simulink model "lib_testValidity"  (R2018b)
settings: Solver=VariableStepAuto  StartTime=0.0  StopTime=tfinal  RelTol=1e-3
model workspace (MAT data in the model file):
  q_init = Simulink.Parameter
  q_init.DataType = 'auto'
  q_init.Dimensions = [0 0]
values from neighbouring files (symbols this model uses):
  Bb = Bb./norm(Bb)    [MEKF_ScriptandSimulink_Test.m]    (also in rfrf.m)
  del_t = tspan(2)-tspan(1)    [MEKF_ScriptandSimulink_Test.m]    (also in rfrf.m)
  q = [q(:,2),q(:,3),q(:,4),q(:,1)]    [MEKF_ScriptandSimulink_Test.m]    (also in rfrf.m)
  Ri = Ri./norm(Ri)    [MEKF_ScriptandSimulink_Test.m]    (also in rfrf.m)
undefined symbols (not defined in the file or in its folder): fswParams
libraries: sharedutil x3, dspmtrx3 x2, MEKF_lib x2, aerolibutil x2
settings Model: Creator=kylle  LastModifiedBy=kylle
settings SolverCC: ConsecutiveZCsStepRelTol=0.00001
settings DataIOCC: ReturnWorkspaceOutputs=on  TimeSaveName=timeoutNew  OutputSaveName=youtNew

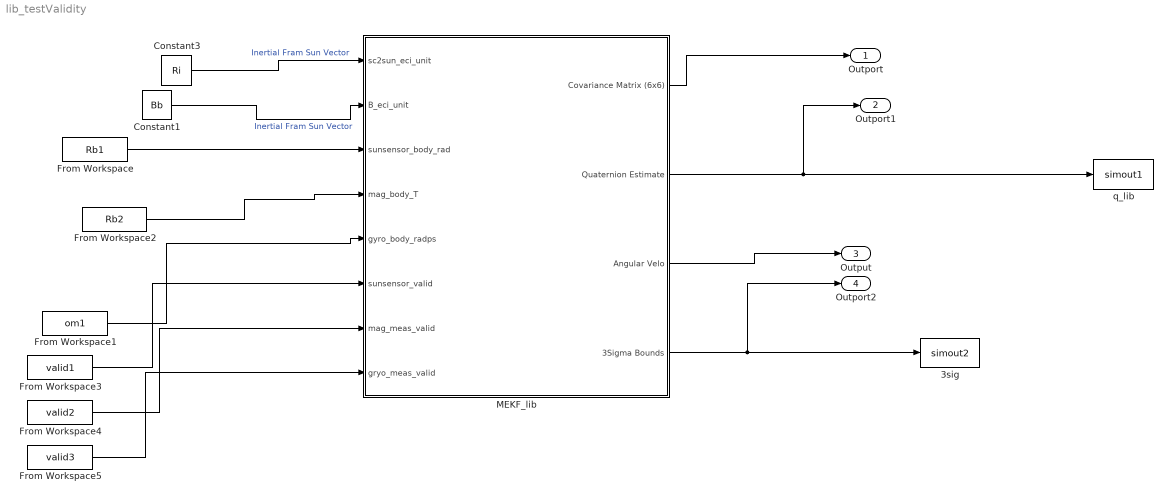
== system lib_testValidity ==
  3sig : ToWorkspace  VariableName=simout2  SaveFormat=Timeseries  SampleTime=-1
  Constant1 : Constant  Value=Bb  VectorParams1D=off
  Constant3 : Constant  Value=Ri  VectorParams1D=off
  From Workspace : FromWorkspace  VariableName=Rb1  SampleTime=del_t
  From Workspace1 : FromWorkspace  VariableName=om1  SampleTime=del_t
  From Workspace2 : FromWorkspace  VariableName=Rb2  SampleTime=del_t
  From Workspace3 : FromWorkspace  VariableName=valid1  SampleTime=del_t
  From Workspace4 : FromWorkspace  VariableName=valid2  SampleTime=del_t
  From Workspace5 : FromWorkspace  VariableName=valid3  SampleTime=del_t
  MEKF_lib : Subsystem  AncestorBlock=MEKF_lib/MEKF_lib
  q_lib : ToWorkspace  VariableName=simout1  SaveFormat=Timeseries  SampleTime=-1
  Outport : Outport
  Outport1 : Outport  Port=2
  Output : Outport  Port=3
  Outport2 : Outport  Port=4
  wires:
  From Workspace1/1 -> MEKF_lib/5(gyro_body_radps)
  MEKF_lib/3("Angular Velo ") -> Output/1
  Constant3/1 -> MEKF_lib/1(sc2sun_eci_unit)  "Inertial Fram Sun Vector"
  MEKF_lib/1(Covariance Matrix (6x6)) -> Outport/1
  Constant1/1 -> MEKF_lib/2(B_eci_unit)  "Inertial Fram Sun Vector"
  From Workspace/1 -> MEKF_lib/3(sunsensor_body_rad)
  From Workspace2/1 -> MEKF_lib/4(mag_body_T)
  From Workspace3/1 -> MEKF_lib/6(sunsensor_valid)
  From Workspace4/1 -> MEKF_lib/7(mag_meas_valid)
  From Workspace5/1 -> MEKF_lib/8(gryo_meas_valid)
  MEKF_lib/2("Quaternion Estimate ") -> q_lib/1, Outport1/1
  MEKF_lib/4("3Sigma Bounds ") -> 3sig/1, Outport2/1

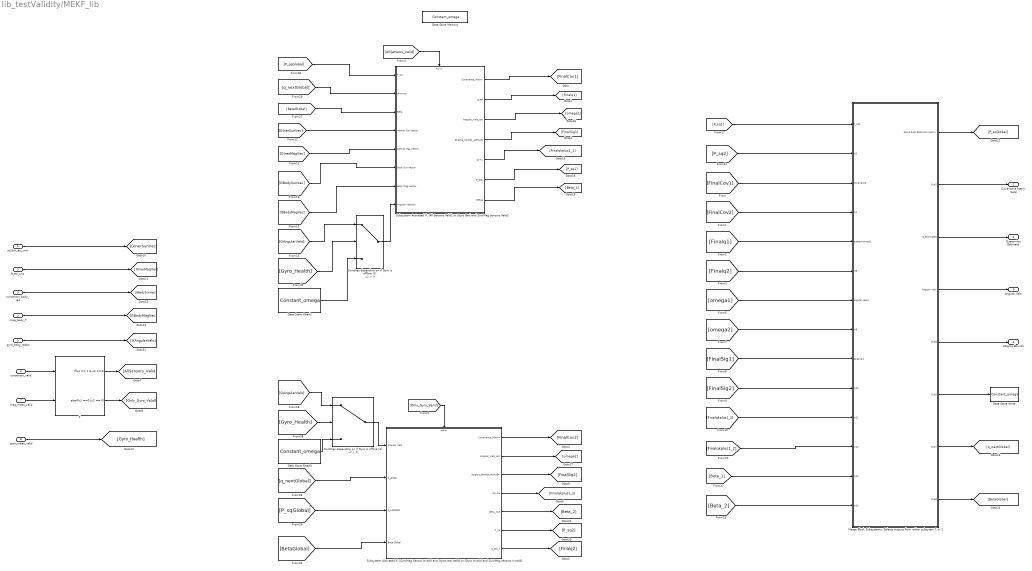
== system lib_testValidity/MEKF_lib ==
  sc2sun_eci_unit : Inport
  B_eci_unit : Inport  Port=2
  sunsensor_body_rad : Inport  Port=3
  mag_body_T : Inport  Port=4
  gyro_body_radps : Inport  Port=5
  sunsensor_valid : Inport  Port=6
  mag_meas_valid : Inport  Port=7
  gryo_meas_valid : Inport  Port=8
  Data Store Memory : DataStoreMemory  DataStoreName=Constant_omega  ReadBeforeWriteMsg=warning  WriteAfterWriteMsg=warning  WriteAfterReadMsg=warning  InitialValue=w0  VectorParams1D=off  ShowAdditionalParam=off
  Data Store Read2 : DataStoreRead  DataStoreName=Constant_omega
  Data Store Read3 : DataStoreRead  DataStoreName=Constant_omega
  Data Store Write : DataStoreWrite  DataStoreName=Constant_omega
  If : If  NumInputs=2  IfExpression=u1 == 1 & u2 ==1  ElseIfExpressions=u1 ==0 |u2 == 0  ShowElse=off
  "Merge Block Subsystems, Selects outputs from either subsytem 1 or 2" : Subsystem
  Subsystem Activated if: [All Sensors Valid] or [Gyro Bad and Sun/Mag sensors Valid] : Subsystem  TreatAsAtomicUnit=on
  Subsystem Activated if: [Sun/Mag Sensor Invalid and Gyros are Valid] or [Gyro Invalid and Sun/Mag sensors Invalid] : Subsystem  TreatAsAtomicUnit=on
  Switches depending on if Gyro is offline (1) : Switch  Criteria=u2 > Threshold
  Switches depending on if Gyro is offline (2) : Switch  Criteria=u2 > Threshold
  Covariance Matrix (6x6) : Outport
  "Quaternion Estimate " : Outport  Port=2
  "Angular Velo " : Outport  Port=3
  "3Sigma Bounds " : Outport  Port=4
  wires:
  [GBodySunVec] -> Subsystem Activated if: [All Sensors Valid] or [Gyro Bad and Sun/Mag sensors Valid]/6(Body Sun Vector)
  [GInerMagVec] -> Subsystem Activated if: [All Sensors Valid] or [Gyro Bad and Sun/Mag sensors Valid]/5(Inertial Mag Vector)
  [GBodyMagVec] -> Subsystem Activated if: [All Sensors Valid] or [Gyro Bad and Sun/Mag sensors Valid]/7(Body Mag Vector)
  Subsystem Activated if: [Sun/Mag Sensor Invalid and Gyros are Valid] or [Gyro Invalid and Sun/Mag sensors Invalid]/4(qk+1a) -> [Finalqkplus1_2]
  Subsystem Activated if: [All Sensors Valid] or [Gyro Bad and Sun/Mag sensors Valid]/2(q_est) -> [Finalq1]
  Subsystem Activated if: [All Sensors Valid] or [Gyro Bad and Sun/Mag sensors Valid]/1(Covariance_Matrix) -> [FinalCov1]
  [Only_Gyro_Valid] -> Subsystem Activated if: [Sun/Mag Sensor Invalid and Gyros are Valid] or [Gyro Invalid and Sun/Mag sensors Invalid]/Action
  Subsystem Activated if: [All Sensors Valid] or [Gyro Bad and Sun/Mag sensors Valid]/4(3sigma_bounds_attitude) -> [FinalSig1]
  Subsystem Activated if: [Sun/Mag Sensor Invalid and Gyros are Valid] or [Gyro Invalid and Sun/Mag sensors Invalid]/7(q_est_k) -> [Finalq2]
  [GInerSunVec] -> Subsystem Activated if: [All Sensors Valid] or [Gyro Bad and Sun/Mag sensors Valid]/4(Inertial Sun Vector)
  Subsystem Activated if: [Sun/Mag Sensor Invalid and Gyros are Valid] or [Gyro Invalid and Sun/Mag sensors Invalid]/1(Covariance_Matrix) -> [FinalCov2]
  [AllSensors_Valid] -> Subsystem Activated if: [All Sensors Valid] or [Gyro Bad and Sun/Mag sensors Valid]/Action
  Subsystem Activated if: [Sun/Mag Sensor Invalid and Gyros are Valid] or [Gyro Invalid and Sun/Mag sensors Invalid]/3(3sigma_bounds_attitude) -> [FinalSig2]
  [q_nextGlobal] -> Subsystem Activated if: [Sun/Mag Sensor Invalid and Gyros are Valid] or [Gyro Invalid and Sun/Mag sensors Invalid]/2(q_global)
  Subsystem Activated if: [All Sensors Valid] or [Gyro Bad and Sun/Mag sensors Valid]/5(qk+1) -> [Finalqkplus1_1]
  [P_sqGlobal] -> Subsystem Activated if: [Sun/Mag Sensor Invalid and Gyros are Valid] or [Gyro Invalid and Sun/Mag sensors Invalid]/3(P_sqGlobal)
  [BetaGlobal] -> Subsystem Activated if: [Sun/Mag Sensor Invalid and Gyros are Valid] or [Gyro Invalid and Sun/Mag sensors Invalid]/4(Beta Global)
  [BetaGlobal] -> Subsystem Activated if: [All Sensors Valid] or [Gyro Bad and Sun/Mag sensors Valid]/3(Beta)
  Subsystem Activated if: [All Sensors Valid] or [Gyro Bad and Sun/Mag sensors Valid]/3(Angular_Velo_est) -> [omega1]
  Subsystem Activated if: [All Sensors Valid] or [Gyro Bad and Sun/Mag sensors Valid]/6("P_Sqa ") -> [P_sq1]
  Subsystem Activated if: [All Sensors Valid] or [Gyro Bad and Sun/Mag sensors Valid]/7(Betaa) -> [Beta_1]
  Subsystem Activated if: [Sun/Mag Sensor Invalid and Gyros are Valid] or [Gyro Invalid and Sun/Mag sensors Invalid]/6(P_sq) -> [P_sq2]
  Subsystem Activated if: [Sun/Mag Sensor Invalid and Gyros are Valid] or [Gyro Invalid and Sun/Mag sensors Invalid]/5(Beta_Out) -> [Beta_2]
  Subsystem Activated if: [Sun/Mag Sensor Invalid and Gyros are Valid] or [Gyro Invalid and Sun/Mag sensors Invalid]/2(Angular_Velo_est) -> [omega2]
  [q_nextGlobal] -> Subsystem Activated if: [All Sensors Valid] or [Gyro Bad and Sun/Mag sensors Valid]/2(qkminus)
  [P_sqGlobal] -> Subsystem Activated if: [All Sensors Valid] or [Gyro Bad and Sun/Mag sensors Valid]/1(P_sq)
  If/1 -> [AllSensors_Valid]
  If/2 -> [Only_Gyro_Valid]
  [GAngularVelo] -> Switches depending on if Gyro is offline (1)/1
  [Gyro_Health] -> Switches depending on if Gyro is offline (1)/2
  Data Store Read2/1 -> Switches depending on if Gyro is offline (1)/3
  Switches depending on if Gyro is offline (1)/1 -> Subsystem Activated if: [All Sensors Valid] or [Gyro Bad and Sun/Mag sensors Valid]/8(Angular Velocity)
  [Gyro_Health] -> Switches depending on if Gyro is offline (2)/2
  [GAngularVelo] -> Switches depending on if Gyro is offline (2)/1
  Data Store Read3/1 -> Switches depending on if Gyro is offline (2)/3
  Switches depending on if Gyro is offline (2)/1 -> Subsystem Activated if: [Sun/Mag Sensor Invalid and Gyros are Valid] or [Gyro Invalid and Sun/Mag sensors Invalid]/1(Angular Velo)
  [P_sq1] -> "Merge Block Subsystems, Selects outputs from either subsytem 1 or 2"/1(P_sq1)
  [P_sq2] -> "Merge Block Subsystems, Selects outputs from either subsytem 1 or 2"/2(In2)
  [FinalCov1] -> "Merge Block Subsystems, Selects outputs from either subsytem 1 or 2"/3(covariance)
  [FinalCov2] -> "Merge Block Subsystems, Selects outputs from either subsytem 1 or 2"/4(In4)
  [Finalq1] -> "Merge Block Subsystems, Selects outputs from either subsytem 1 or 2"/5(quaternion est1)
  [Finalq2] -> "Merge Block Subsystems, Selects outputs from either subsytem 1 or 2"/6(In6)
  [omega1] -> "Merge Block Subsystems, Selects outputs from either subsytem 1 or 2"/7(angular velo1)
  [omega2] -> "Merge Block Subsystems, Selects outputs from either subsytem 1 or 2"/8(In8)
  [FinalSig1] -> "Merge Block Subsystems, Selects outputs from either subsytem 1 or 2"/9(3sigma 1)
  [FinalSig2] -> "Merge Block Subsystems, Selects outputs from either subsytem 1 or 2"/10(In10)
  [Finalqkplus1_1] -> "Merge Block Subsystems, Selects outputs from either subsytem 1 or 2"/11(In11)
  [Finalqkplus1_2] -> "Merge Block Subsystems, Selects outputs from either subsytem 1 or 2"/12(In12)
  [Beta_1] -> "Merge Block Subsystems, Selects outputs from either subsytem 1 or 2"/13(In13)
  [Beta_2] -> "Merge Block Subsystems, Selects outputs from either subsytem 1 or 2"/14(In14)
  "Merge Block Subsystems, Selects outputs from either subsytem 1 or 2"/1(Squre Root State Cov Matrix) -> [P_sqGlobal]
  "Merge Block Subsystems, Selects outputs from either subsytem 1 or 2"/2(Out2) -> Covariance Matrix (6x6)/1
  "Merge Block Subsystems, Selects outputs from either subsytem 1 or 2"/3(q_estimated) -> "Quaternion Estimate "/1
  "Merge Block Subsystems, Selects outputs from either subsytem 1 or 2"/4(Angular Velo) -> "Angular Velo "/1
  "Merge Block Subsystems, Selects outputs from either subsytem 1 or 2"/6(Out5) -> Data Store Write/1
  "Merge Block Subsystems, Selects outputs from either subsytem 1 or 2"/5(Out6) -> "3Sigma Bounds "/1
  "Merge Block Subsystems, Selects outputs from either subsytem 1 or 2"/7(Out7) -> [q_nextGlobal]
  "Merge Block Subsystems, Selects outputs from either subsytem 1 or 2"/8(Out8) -> [BetaGlobal]
  sc2sun_eci_unit/1 -> [GInerSunVec]
  sunsensor_body_rad/1 -> [GBodySunVec]
  sunsensor_valid/1 -> If/1
  mag_meas_valid/1 -> If/2
  gryo_meas_valid/1 -> [Gyro_Health]
  B_eci_unit/1 -> [GInerMagVec]
  mag_body_T/1 -> [GBodyMagVec]
  gyro_body_radps/1 -> [GAngularVelo]

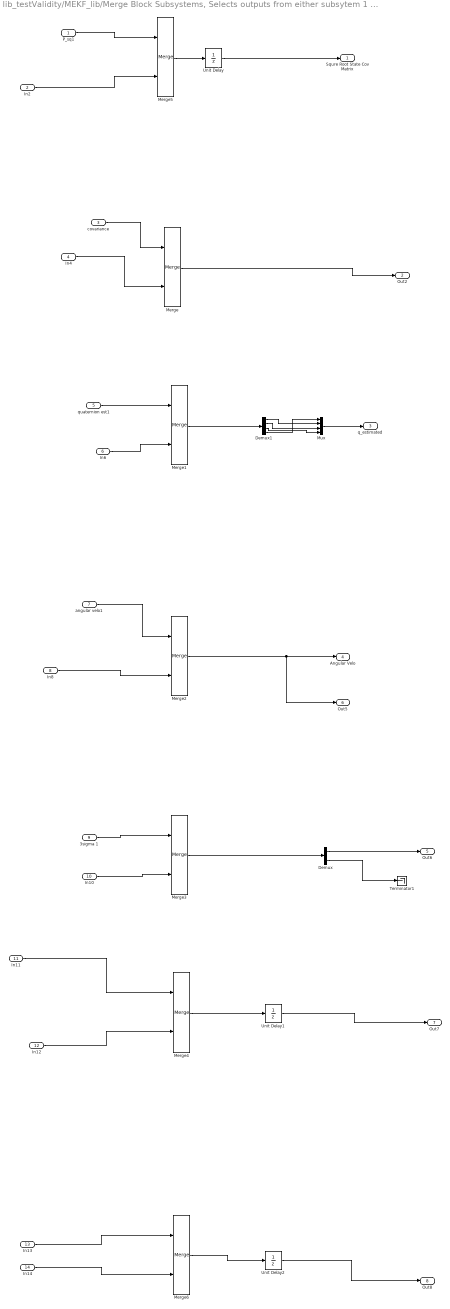
== system lib_testValidity/MEKF_lib/Merge Block Subsystems, Selects outputs from either subsytem 1 or 2 ==
  P_sq1 : Inport
  In2 : Inport  Port=2
  covariance : Inport  Port=3
  In4 : Inport  Port=4
  quaternion est1 : Inport  Port=5
  In6 : Inport  Port=6
  angular velo1 : Inport  Port=7
  In8 : Inport  Port=8
  3sigma 1 : Inport  Port=9
  In10 : Inport  Port=10
  In11 : Inport  Port=11
  In12 : Inport  Port=12
  In13 : Inport  Port=13
  In14 : Inport  Port=14
  Demux : Demux  Outputs=2
  Demux1 : Demux
  Merge{,1..6} (7 alike) : Merge
  Mux : Mux
  Terminator1 : Terminator
  Unit Delay : UnitDelay  InitialCondition=fswParams.estimation.ic.P_sq_init  SampleTime=-1
  Unit Delay1 : UnitDelay  InitialCondition=fswParams.estimation.ic.quat_est_init  SampleTime=-1
  Unit Delay2 : UnitDelay  InitialCondition=fswParams.estimation.ic.Beta_init  SampleTime=-1
  Squre Root State Cov Matrix : Outport
  Out2 : Outport  Port=2
  q_estimated : Outport  Port=3
  Angular Velo : Outport  Port=4
  Out6 : Outport  Port=5
  Out5 : Outport  Port=6
  Out7 : Outport  Port=7
  Out8 : Outport  Port=8
  wires:
  Merge3/1 -> Demux/1
  Merge2/1 -> Out5/1, Angular Velo/1
  Unit Delay1/1 -> Out7/1
  Demux/2 -> Terminator1/1
  Merge6/1 -> Unit Delay2/1
  3sigma 1/1 -> Merge3/1
  quaternion est1/1 -> Merge1/1
  In14/1 -> Merge6/2
  angular velo1/1 -> Merge2/1
  In11/1 -> Merge4/1
  Merge5/1 -> Unit Delay/1
  In10/1 -> Merge3/2
  In2/1 -> Merge5/2
  covariance/1 -> Merge/1
  Merge4/1 -> Unit Delay1/1
  In4/1 -> Merge/2
  Demux/1 -> Out6/1
  In13/1 -> Merge6/1
  Merge/1 -> Out2/1
  In6/1 -> Merge1/2
  In8/1 -> Merge2/2
  In12/1 -> Merge4/2
  P_sq1/1 -> Merge5/1
  Unit Delay2/1 -> Out8/1
  Unit Delay/1 -> Squre Root State Cov Matrix/1
  Merge1/1 -> Demux1/1
  Demux1/4 -> Mux/1
  Demux1/1 -> Mux/2
  Demux1/2 -> Mux/3
  Demux1/3 -> Mux/4
  Mux/1 -> q_estimated/1

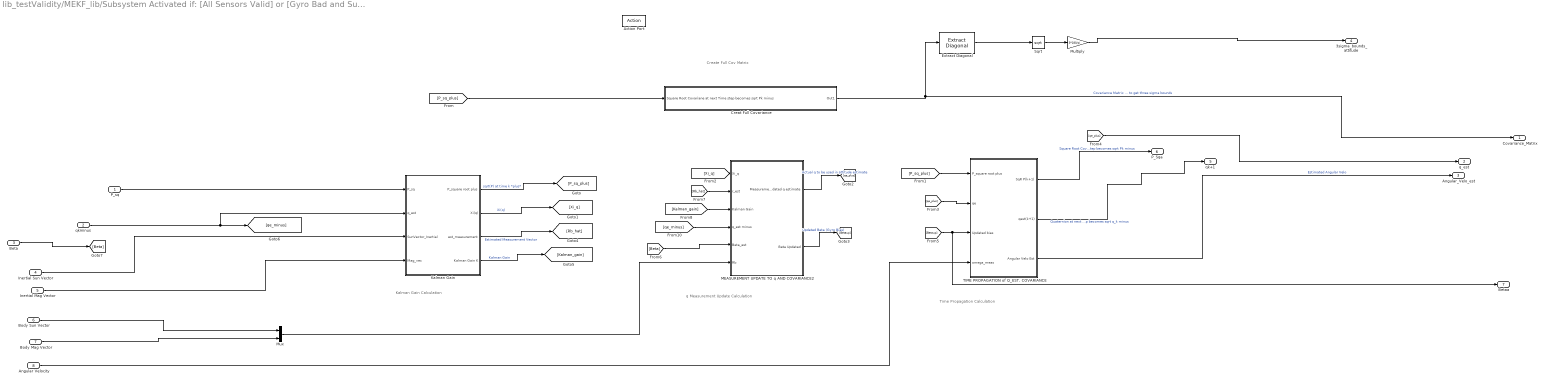
== system lib_testValidity/MEKF_lib/Subsystem Activated if: [All Sensors Valid] or [Gyro Bad and Sun//Mag sensors Valid] ==
  note: Kalman Gain Calculation
  note: Time Propagation Calculation
  note: Create Full Cov Matrix
  note: q Measurement Update Calculation
  P_sq : Inport
  qkminus : Inport  Port=2
  Beta : Inport  Port=3
  Inertial Sun Vector : Inport  Port=4
  Inertial Mag Vector : Inport  Port=5
  Body Sun Vector : Inport  Port=6
  Body Mag Vector : Inport  Port=7
  Angular Velocity : Inport  Port=8
  Action Port : ActionPort  ActionType=then
  Creat Full Covariance : Subsystem  AncestorBlock=MEKF_LibraryR2018b/Multiplicative Extended Kalman Filter/Creat Full Covariance
  Extract Diagonal : dspmtrx3/Extract Diagonal
      settings: SourceProductName=DSP System Toolbox  SourceProductBaseCode=DS
  Kalman Gain : Subsystem  AncestorBlock=MEKF_LibraryR2018b/Multiplicative Extended Kalman Filter/Kalman Gain
  MEASUREMENT UPDATE TO q AND COVARIANCE2 : Subsystem  AncestorBlock=MEKF_LibraryR2018b/Multiplicative Extended Kalman Filter/MEASUREMENT UPDATE TO q AND COVARIANCE2
  Multiply : Gain  Gain=3*180/pi
  Mux : Mux  Inputs=2
  Sqrt : Sqrt  SaturateOnIntegerOverflow=on
  "TIME PROPAGATION of Q_EST, COVARIANCE" : Subsystem  AncestorBlock=MEKF_Library/Multiplicative Extended Kalman Filter/TIME PROPAGATION of Q_EST, COVARIANCE
  Covariance_Matrix : Outport
  q_est : Outport  Port=2
  Angular_Velo_est : Outport  Port=3
  3sigma_bounds_attitude : Outport  Port=4
  qk+1 : Outport  Port=5
  "P_Sqa " : Outport  Port=6
  Betaa : Outport  Port=7
  wires:
  Inertial Sun Vector/1 -> Kalman Gain/3(SunVector_Inertial)
  [qe_plus] -> q_est/1
  "TIME PROPAGATION of Q_EST, COVARIANCE"/2(qest(k+1)) -> qk+1/1  "Quaternion at next Time step becomes sqrt q_k minus"
  "TIME PROPAGATION of Q_EST, COVARIANCE"/3(Angular Velo Est) -> Angular_Velo_est/1  "Estimated Angular Velo"
  Creat Full Covariance/1(Out1) -> Covariance_Matrix/1, Extract Diagonal/1  "Covariance Matrix from which to get three sigma bounds"
  qkminus/1 -> Kalman Gain/2(q_est), [qe_minus]
  Extract Diagonal/1 -> Sqrt/1
  Angular Velocity/1 -> "TIME PROPAGATION of Q_EST, COVARIANCE"/4(omega_meas)
  P_sq/1 -> Kalman Gain/1(P_sq)
  [qe_plus] -> "TIME PROPAGATION of Q_EST, COVARIANCE"/2(qe)
  MEASUREMENT UPDATE TO q AND COVARIANCE2/2(Beta Updated) -> [Betaup]  "Updated Beta (Gyro Bias)"
  [Rb_hat] -> MEASUREMENT UPDATE TO q AND COVARIANCE2/2(r_est)
  "TIME PROPAGATION of Q_EST, COVARIANCE"/1(SqR P(k+1)) -> "P_Sqa "/1  "Square Root Covariane at next Time step becomes sqrt Pk minus"
  Kalman Gain/1(P_square root plus) -> [P_sq_plus]  "sqrt(P) at time k *plus*"
  Kalman Gain/4(Kalman Gain K) -> [Kalman_gain]  "Kalman Gain"
  [qe_minus] -> MEASUREMENT UPDATE TO q AND COVARIANCE2/4(q_est minus)
  Kalman Gain/2(Xi(q)) -> [Xi_q]  "Xi(q)"
  Sqrt/1 -> Multiply/1
  [P_sq_plus] -> Creat Full Covariance/1(Square Root Covariane at next Time step becomes sqrt Pk minus)
  [Betaup] -> Betaa/1, "TIME PROPAGATION of Q_EST, COVARIANCE"/3(Updated bias)
  [Beta] -> MEASUREMENT UPDATE TO q AND COVARIANCE2/5(Beta_est)
  MEASUREMENT UPDATE TO q AND COVARIANCE2/1(Measurement updated q estimate) -> [qe_plus]  "Actual q to be used in attitude estimate"
  [P_sq_plus] -> "TIME PROPAGATION of Q_EST, COVARIANCE"/1(P_square root plus)
  Kalman Gain/3(est_measurement) -> [Rb_hat]  "Estimated Measurement Vector"
  [Xi_q] -> MEASUREMENT UPDATE TO q AND COVARIANCE2/1(Xi_q)
  [Kalman_gain] -> MEASUREMENT UPDATE TO q AND COVARIANCE2/3(Kalman Gain)
  Inertial Mag Vector/1 -> Kalman Gain/4("Mag_vec ")
  Body Sun Vector/1 -> Mux/1
  Body Mag Vector/1 -> Mux/2
  Mux/1 -> MEASUREMENT UPDATE TO q AND COVARIANCE2/6(Rb)
  Multiply/1 -> 3sigma_bounds_attitude/1
  Beta/1 -> [Beta]

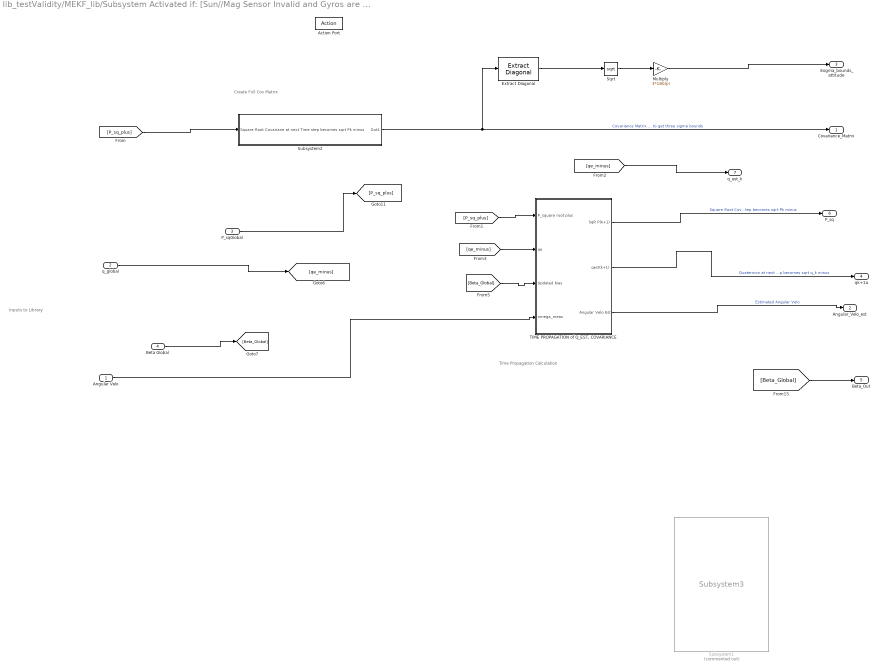
== system lib_testValidity/MEKF_lib/Subsystem Activated if: [Sun//Mag Sensor Invalid and Gyros are Valid] or [Gyro Invalid and Sun//Mag sensors Invalid] ==
  note: Create Full Cov Matrix
  note: Inputs to Library
  note: Time Propagation Calculation
  Angular Velo : Inport
  q_global : Inport  Port=2
  P_sqGlobal : Inport  Port=3
  Beta Global : Inport  Port=4
  Action Port : ActionPort  ActionType=elseif
  Extract Diagonal : dspmtrx3/Extract Diagonal
      settings: SourceProductName=DSP System Toolbox  SourceProductBaseCode=DS
  Multiply : Gain  Gain=3*180/pi
  Sqrt : Sqrt  SaturateOnIntegerOverflow=on
  Subsystem1 : MEKF_lib/MEKF with Validity Check/Subsystem Activated if: [Sun//Mag Sensor Invalid and Gyros are Valid] or [Gyro Invalid and Sun//Mag sensors Invalid]/Subsystem3  Commented=on  SystemSampleTime=-1  SSRTWFcnClass=[]
  Subsystem2 : Subsystem
  "TIME PROPAGATION of Q_EST, COVARIANCE" : Subsystem  AncestorBlock=|
      | MEKF_SensorCheck_Lib2018/MEKF with Validity Check/Subsystem Activated if: [All Sensors Valid]
      | or
      | [Gyro Bad and Sun//Mag sensors Valid]/TIME PROPAGATION of Q_EST, COVARIANCE
  Covariance_Matrix : Outport
  Angular_Velo_est : Outport  Port=2
  3sigma_bounds_attitude : Outport  Port=3
  qk+1a : Outport  Port=4
  Beta_Out : Outport  Port=5
  P_sq : Outport  Port=6
  q_est_k : Outport  Port=7
  wires:
  P_sqGlobal/1 -> [P_sq_plus]
  [qe_minus] -> "TIME PROPAGATION of Q_EST, COVARIANCE"/2(qe)
  "TIME PROPAGATION of Q_EST, COVARIANCE"/2(qest(k+1)) -> qk+1a/1  "Quaternion at next Time step becomes sqrt q_k minus"
  Sqrt/1 -> Multiply/1
  Subsystem2/1(Out1) -> Covariance_Matrix/1, Extract Diagonal/1  "Covariance Matrix from which to get three sigma bounds"
  "TIME PROPAGATION of Q_EST, COVARIANCE"/3(Angular Velo Est) -> Angular_Velo_est/1  "Estimated Angular Velo"
  [P_sq_plus] -> Subsystem2/1(Square Root Covariane at next Time step becomes sqrt Pk minus)
  [P_sq_plus] -> "TIME PROPAGATION of Q_EST, COVARIANCE"/1(P_square root plus)
  [Beta_Global] -> "TIME PROPAGATION of Q_EST, COVARIANCE"/3(Updated bias)
  Extract Diagonal/1 -> Sqrt/1
  q_global/1 -> [qe_minus]
  Angular Velo/1 -> "TIME PROPAGATION of Q_EST, COVARIANCE"/4(omega_meas)
  Multiply/1 -> 3sigma_bounds_attitude/1
  "TIME PROPAGATION of Q_EST, COVARIANCE"/1(SqR P(k+1)) -> P_sq/1  "Square Root Covariane at next Time step becomes sqrt Pk minus"
  Beta Global/1 -> [Beta_Global]
  [Beta_Global] -> Beta_Out/1
  [qe_minus] -> q_est_k/1

== system lib_testValidity/MEKF_lib/Subsystem Activated if: [All Sensors Valid] or [Gyro Bad and Sun//Mag sensors Valid]/Creat Full Covariance ==
  Square Root Covariane at next Time step becomes sqrt Pk minus : Inport
  Matrix Multiply : Product  Multiplication=Matrix(*)
  Transpose : Math  Operator=transpose  SaturateOnIntegerOverflow=on
  Out1 : Outport
  wires:
  Square Root Covariane at next Time step becomes sqrt Pk minus/1 -> Transpose/1, Matrix Multiply/1
  Transpose/1 -> Matrix Multiply/2
  Matrix Multiply/1 -> Out1/1

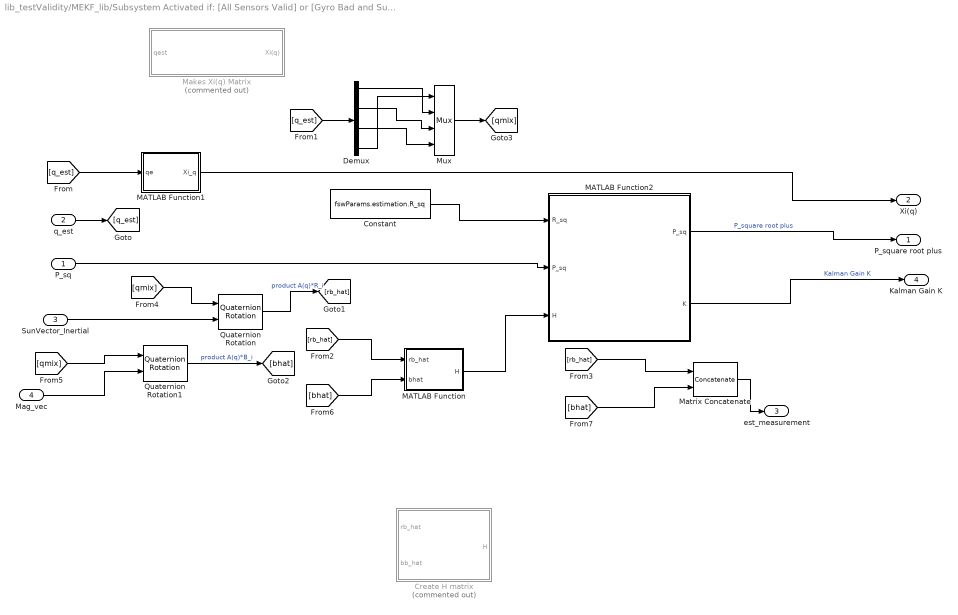
== system lib_testValidity/MEKF_lib/Subsystem Activated if: [All Sensors Valid] or [Gyro Bad and Sun//Mag sensors Valid]/Kalman Gain ==
  P_sq : Inport
  q_est : Inport  Port=2
  SunVector_Inertial : Inport  Port=3
  "Mag_vec " : Inport  Port=4
  Constant : Constant  Value=fswParams.estimation.R_sq  VectorParams1D=off
  Create H matrix : Subsystem  Commented=on
  Demux : Demux
  MATLAB Function : MATLAB Function  TreatAsAtomicUnit=on
  MATLAB Function1 : MATLAB Function  TreatAsAtomicUnit=on
  MATLAB Function2 : MATLAB Function  TreatAsAtomicUnit=on
  Makes Xi(q) Matrix : Subsystem  Commented=on
  Matrix Concatenate : Concatenate  Mode=Multidimensional array
  Mux : Mux
  Quaternion Rotation : aerolibutil/Quaternion Rotation
  Quaternion Rotation1 : aerolibutil/Quaternion Rotation
  P_square root plus : Outport
  Xi(q) : Outport  Port=2
  est_measurement : Outport  Port=3
  Kalman Gain K : Outport  Port=4
  wires:
  P_sq/1 -> MATLAB Function2/2("P_sq ")
  MATLAB Function2/2(K) -> Kalman Gain K/1  "Kalman Gain K"
  SunVector_Inertial/1 -> Quaternion Rotation/2
  Constant/1 -> MATLAB Function2/1(R_sq)
  MATLAB Function2/1(P_sq) -> P_square root plus/1  "P_square root plus"
  Demux/1 -> Mux/2
  Demux/2 -> Mux/3
  Demux/3 -> Mux/4
  Demux/4 -> Mux/1
  q_est/1 -> [q_est]
  [q_est] -> Demux/1
  Quaternion Rotation/1 -> [rb_hat]  "product A(q)*R_i"
  "Mag_vec "/1 -> Quaternion Rotation1/2
  Quaternion Rotation1/1 -> [bhat]  "product A(q)*B_i"
  Mux/1 -> [qmix]
  [qmix] -> Quaternion Rotation1/1
  [qmix] -> Quaternion Rotation/1
  [rb_hat] -> Matrix Concatenate/1
  [bhat] -> Matrix Concatenate/2
  Matrix Concatenate/1 -> est_measurement/1
  [rb_hat] -> MATLAB Function/1(rb_hat)
  [bhat] -> MATLAB Function/2(bhat)
  MATLAB Function/1(H) -> MATLAB Function2/3(H)
  [q_est] -> MATLAB Function1/1(qe)
  MATLAB Function1/1(Xi_q) -> Xi(q)/1

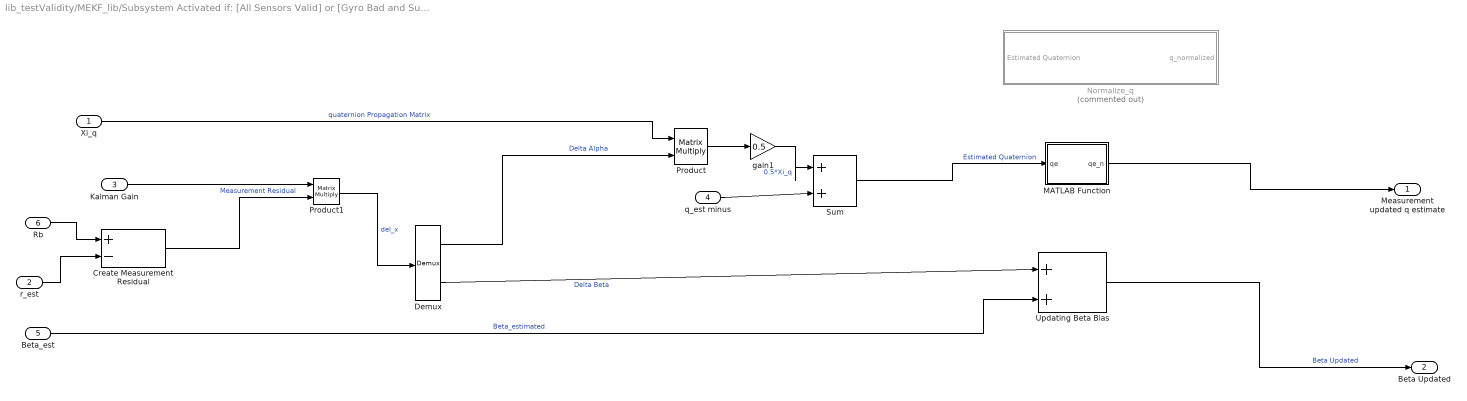
== system lib_testValidity/MEKF_lib/Subsystem Activated if: [All Sensors Valid] or [Gyro Bad and Sun//Mag sensors Valid]/MEASUREMENT UPDATE TO q AND COVARIANCE2 ==
  Xi_q : Inport
  r_est : Inport  Port=2
  Kalman Gain : Inport  Port=3
  q_est minus : Inport  Port=4
  Beta_est : Inport  Port=5
  Rb : Inport  Port=6
  Create Measurement Residual : Sum  Inputs=+-
  Demux : Demux  Outputs=2
  MATLAB Function : MATLAB Function  TreatAsAtomicUnit=on
  Normalize_q : Subsystem  Commented=on
  Product : Product  Inputs=**  Multiplication=Matrix(*)
  Product1 : Product  Multiplication=Matrix(*)
  Sum : Sum  Inputs=|++
  "Updating Beta Bias " : Sum  Inputs=|++
  gain1 : Gain  Gain=0.5
  Measurement updated q estimate : Outport
  Beta Updated : Outport  Port=2
  wires:
  Demux/1 -> Product/2  "Delta Alpha"
  Demux/2 -> "Updating Beta Bias "/1  "Delta Beta"
  Product1/1 -> Demux/1  "del_x"
  r_est/1 -> Create Measurement Residual/2
  Create Measurement Residual/1 -> Product1/2  "Measurement Residual"
  "Updating Beta Bias "/1 -> Beta Updated/1  "Beta Updated"
  Beta_est/1 -> "Updating Beta Bias "/2  "Beta_estimated"
  q_est minus/1 -> Sum/2
  Kalman Gain/1 -> Product1/1
  Rb/1 -> Create Measurement Residual/1
  Xi_q/1 -> Product/1  "quaternion Propagation Matrix"
  Product/1 -> gain1/1
  gain1/1 -> Sum/1  "0.5*Xi_q"
  Sum/1 -> MATLAB Function/1(qe)  "Estimated Quaternion"
  MATLAB Function/1(qe_n) -> Measurement updated q estimate/1

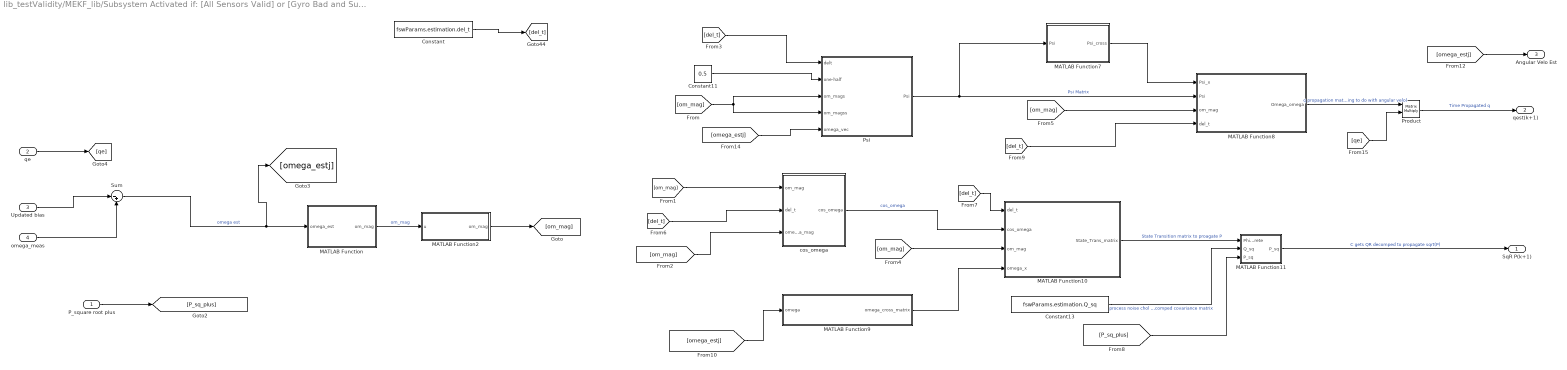
== system lib_testValidity/MEKF_lib/Subsystem Activated if: [All Sensors Valid] or [Gyro Bad and Sun//Mag sensors Valid]/TIME PROPAGATION of Q_EST, COVARIANCE ==
  P_square root plus : Inport
  qe : Inport  Port=2
  Updated bias : Inport  Port=3
  omega_meas : Inport  Port=4
  Constant : Constant  Value=fswParams.estimation.del_t
  Constant11 : Constant  Value=0.5
  Constant13 : Constant  Value=fswParams.estimation.Q_sq  VectorParams1D=off
  MATLAB Function : MATLAB Function  TreatAsAtomicUnit=on
  MATLAB Function10 : MATLAB Function  TreatAsAtomicUnit=on
  MATLAB Function11 : MATLAB Function  TreatAsAtomicUnit=on
  MATLAB Function2 : MATLAB Function  TreatAsAtomicUnit=on
  MATLAB Function7 : MATLAB Function  TreatAsAtomicUnit=on
  MATLAB Function8 : MATLAB Function  TreatAsAtomicUnit=on
  MATLAB Function9 : MATLAB Function  TreatAsAtomicUnit=on
  Product : Product  Multiplication=Matrix(*)
  Psi : Subsystem
  Sum : Sum  Inputs=|-+
  cos_omega : Subsystem
  SqR P(k+1) : Outport
  qest(k+1) : Outport  Port=2
  Angular Velo Est : Outport  Port=3
  wires:
  [del_t] -> MATLAB Function8/4(del_t)
  MATLAB Function7/1(Psi_cross) -> MATLAB Function8/1(Psi_x)
  MATLAB Function11/1(P_sq) -> SqR P(k+1)/1  "C gets QR decomped to propagate sqrt(P)"
  MATLAB Function8/1(Omega_omega) -> Product/1  "q propagation matrix (nothing to do with angular velo)"
  MATLAB Function9/1(omega_cross_matrix) -> MATLAB Function10/4(omega_x)
  MATLAB Function10/1(State_Trans_matrix) -> MATLAB Function11/1(Phi_discrete)  "State Transition matrix to proagate P"
  Product/1 -> qest(k+1)/1  "Time Propagated q"
  Constant13/1 -> MATLAB Function11/2(Q_sq)  "process noise chol decomped covariance matrix"
  omega_meas/1 -> Sum/2
  Updated bias/1 -> Sum/1
  MATLAB Function/1(om_mag) -> MATLAB Function2/1(u)  "om_mag"
  [om_mag] -> MATLAB Function10/3(om_mag)
  [om_mag] -> MATLAB Function8/3(om_mag)
  [del_t] -> MATLAB Function10/1(del_t)
  P_square root plus/1 -> [P_sq_plus]
  [P_sq_plus] -> MATLAB Function11/3("P_sq ")
  [omega_estj] -> MATLAB Function9/1(omega)
  [omega_estj] -> Angular Velo Est/1
  qe/1 -> [qe]
  [qe] -> Product/2
  [om_mag] -> cos_omega/1(om_mag)
  [om_mag] -> cos_omega/3(omega_mag)
  cos_omega/1(cos_omega) -> MATLAB Function10/2(cos_omega)  "cos_omega"
  Psi/1(Psi) -> MATLAB Function8/2(Psi), MATLAB Function7/1(Psi)  "Psi Matrix"
  [del_t] -> Psi/1(delt)
  Constant11/1 -> Psi/2(one-half)
  [omega_estj] -> Psi/5(omega_vec)
  [om_mag] -> Psi/3(om_mags), Psi/4(om_magss)
  Sum/1 -> [omega_estj], MATLAB Function/1(omega_est)  "omega est"
  [del_t] -> cos_omega/2(del_t)
  Constant/1 -> [del_t]
  MATLAB Function2/1(om_mag) -> [om_mag]

== system lib_testValidity/MEKF_lib/Subsystem Activated if: [Sun//Mag Sensor Invalid and Gyros are Valid] or [Gyro Invalid and Sun//Mag sensors Invalid]/Subsystem2 ==
  Square Root Covariane at next Time step becomes sqrt Pk minus : Inport
  Matrix Multiply : Product  Multiplication=Matrix(*)
  Transpose : Math  Operator=transpose  SaturateOnIntegerOverflow=on
  Out1 : Outport
  wires:
  Matrix Multiply/1 -> Out1/1
  Transpose/1 -> Matrix Multiply/2
  Square Root Covariane at next Time step becomes sqrt Pk minus/1 -> Transpose/1, Matrix Multiply/1

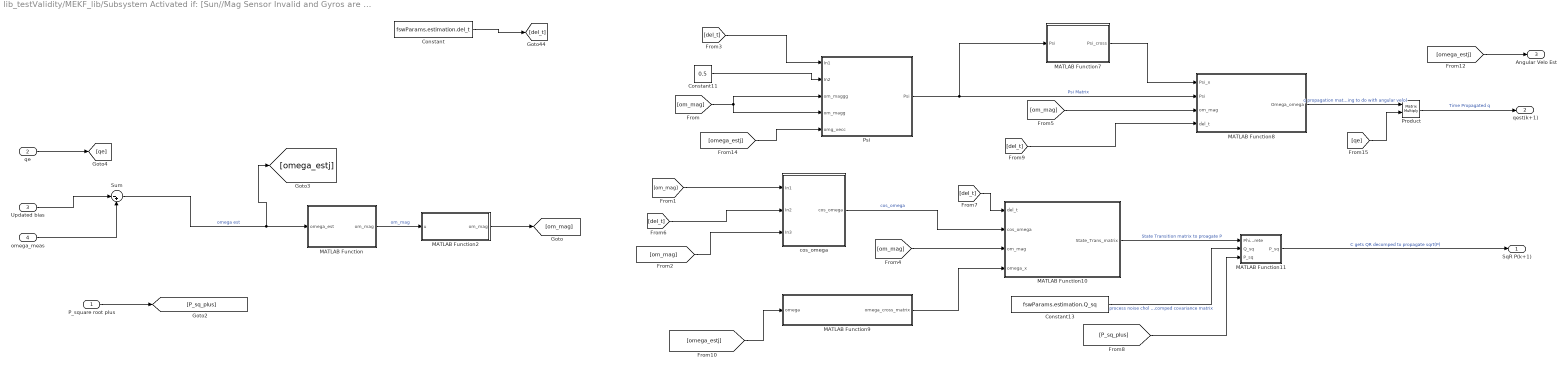
== system lib_testValidity/MEKF_lib/Subsystem Activated if: [Sun//Mag Sensor Invalid and Gyros are Valid] or [Gyro Invalid and Sun//Mag sensors Invalid]/TIME PROPAGATION of Q_EST, COVARIANCE ==
  P_square root plus : Inport
  qe : Inport  Port=2
  Updated bias : Inport  Port=3
  omega_meas : Inport  Port=4
  Constant : Constant  Value=fswParams.estimation.del_t
  Constant11 : Constant  Value=0.5
  Constant13 : Constant  Value=fswParams.estimation.Q_sq  VectorParams1D=off
  MATLAB Function : MATLAB Function  TreatAsAtomicUnit=on
  MATLAB Function10 : MATLAB Function  TreatAsAtomicUnit=on
  MATLAB Function11 : MATLAB Function  TreatAsAtomicUnit=on
  MATLAB Function2 : MATLAB Function  TreatAsAtomicUnit=on
  MATLAB Function7 : MATLAB Function  TreatAsAtomicUnit=on
  MATLAB Function8 : MATLAB Function  TreatAsAtomicUnit=on
  MATLAB Function9 : MATLAB Function  TreatAsAtomicUnit=on
  Product : Product  Multiplication=Matrix(*)
  Psi : Subsystem
  Sum : Sum  Inputs=|-+
  cos_omega : Subsystem
  SqR P(k+1) : Outport
  qest(k+1) : Outport  Port=2
  Angular Velo Est : Outport  Port=3
  wires:
  MATLAB Function2/1(om_mag) -> [om_mag]
  Constant/1 -> [del_t]
  [del_t] -> cos_omega/2(In2)
  Sum/1 -> MATLAB Function/1(omega_est), [omega_estj]  "omega est"
  [om_mag] -> Psi/4(om_magg), Psi/3(om_maggg)
  [omega_estj] -> Psi/5(omg_vecc)
  Constant11/1 -> Psi/2(In2)
  [del_t] -> Psi/1(In1)
  Psi/1(Psi) -> MATLAB Function7/1(Psi), MATLAB Function8/2(Psi)  "Psi Matrix"
  cos_omega/1(cos_omega) -> MATLAB Function10/2(cos_omega)  "cos_omega"
  [om_mag] -> cos_omega/3(In3)
  [om_mag] -> cos_omega/1(In1)
  [qe] -> Product/2
  qe/1 -> [qe]
  [omega_estj] -> Angular Velo Est/1
  [omega_estj] -> MATLAB Function9/1(omega)
  [P_sq_plus] -> MATLAB Function11/3("P_sq ")
  P_square root plus/1 -> [P_sq_plus]
  [del_t] -> MATLAB Function10/1(del_t)
  [om_mag] -> MATLAB Function8/3(om_mag)
  [om_mag] -> MATLAB Function10/3(om_mag)
  MATLAB Function/1(om_mag) -> MATLAB Function2/1(u)  "om_mag"
  Updated bias/1 -> Sum/1
  omega_meas/1 -> Sum/2
  Constant13/1 -> MATLAB Function11/2(Q_sq)  "process noise chol decomped covariance matrix"
  Product/1 -> qest(k+1)/1  "Time Propagated q"
  MATLAB Function10/1(State_Trans_matrix) -> MATLAB Function11/1(Phi_discrete)  "State Transition matrix to proagate P"
  MATLAB Function9/1(omega_cross_matrix) -> MATLAB Function10/4(omega_x)
  MATLAB Function8/1(Omega_omega) -> Product/1  "q propagation matrix (nothing to do with angular velo)"
  MATLAB Function11/1(P_sq) -> SqR P(k+1)/1  "C gets QR decomped to propagate sqrt(P)"
  MATLAB Function7/1(Psi_cross) -> MATLAB Function8/1(Psi_x)
  [del_t] -> MATLAB Function8/4(del_t)

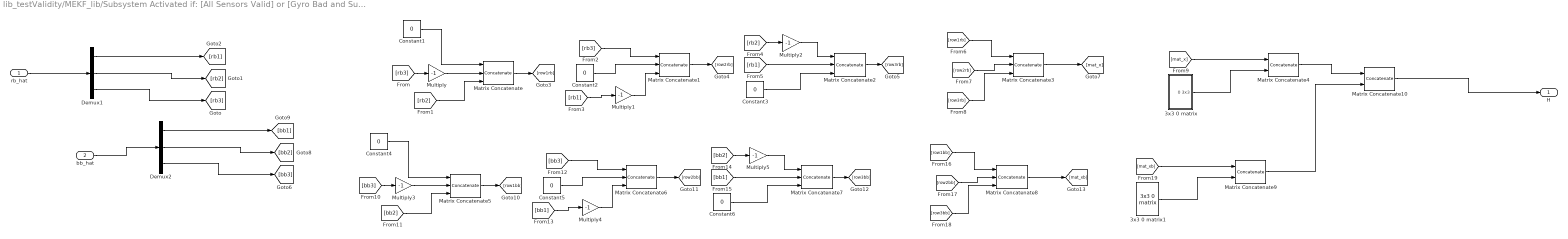
== system lib_testValidity/MEKF_lib/Subsystem Activated if: [All Sensors Valid] or [Gyro Bad and Sun//Mag sensors Valid]/Kalman Gain/Create H matrix ==
  rb_hat : Inport
  bb_hat : Inport  Port=2
  3x3 0 matrix : Subsystem
  3x3 0 matrix1 : MEKF_lib/MEKF_lib/Subsystem Activated if: [All Sensors Valid] or [Gyro Bad and Sun//Mag sensors Valid]/Kalman Gain/Create H matrix/3x3 0 matrix  SystemSampleTime=-1
  Constant{1..6} (6 alike) : Constant  Value=0
  Demux1 : Demux  Outputs=3
  Demux2 : Demux  Outputs=3
  Matrix Concatenate{,1..2,5..7} (6 alike) : Concatenate  NumInputs=3  Mode=Multidimensional array  ConcatenateDimension=2
  Matrix Concatenate10 : Concatenate  Mode=Multidimensional array
  Matrix Concatenate3 : Concatenate  NumInputs=3  Mode=Multidimensional array
  Matrix Concatenate4 : Concatenate  Mode=Multidimensional array  ConcatenateDimension=2
  Matrix Concatenate8 : Concatenate  NumInputs=3  Mode=Multidimensional array
  Matrix Concatenate9 : Concatenate  Mode=Multidimensional array  ConcatenateDimension=2
  Multiply{,1..5} (6 alike) : Gain  Gain=-1
  H : Outport
  wires:
  Matrix Concatenate1/1 -> [row2rb]
  Multiply/1 -> Matrix Concatenate/2
  [mat_x] -> Matrix Concatenate4/1
  Demux1/2 -> [rb2]
  Multiply2/1 -> Matrix Concatenate2/1
  [row3rb] -> Matrix Concatenate3/3
  Matrix Concatenate/1 -> [row1rb]
  Matrix Concatenate2/1 -> [row3rb]
  [rb1] -> Multiply1/1
  [rb3] -> Multiply/1
  Multiply1/1 -> Matrix Concatenate1/3
  Constant3/1 -> Matrix Concatenate2/3
  3x3 0 matrix/1(0 3x3) -> Matrix Concatenate4/2
  [rb2] -> Multiply2/1
  [rb2] -> Matrix Concatenate/3
  [rb3] -> Matrix Concatenate1/1
  [row2rb] -> Matrix Concatenate3/2
  Constant1/1 -> Matrix Concatenate/1
  [row1rb] -> Matrix Concatenate3/1
  Demux1/1 -> [rb1]
  Matrix Concatenate3/1 -> [mat_x]
  Constant2/1 -> Matrix Concatenate1/2
  [rb1] -> Matrix Concatenate2/2
  Demux1/3 -> [rb3]
  rb_hat/1 -> Demux1/1
  Demux2/3 -> [bb3]
  bb_hat/1 -> Demux2/1
  Demux2/1 -> [bb1]
  Demux2/2 -> [bb2]
  Multiply5/1 -> Matrix Concatenate7/1
  [bb1] -> Matrix Concatenate7/2
  Constant4/1 -> Matrix Concatenate5/1
  Multiply3/1 -> Matrix Concatenate5/2
  Constant5/1 -> Matrix Concatenate6/2
  Multiply4/1 -> Matrix Concatenate6/3
  Matrix Concatenate5/1 -> [row1bb]
  [bb1] -> Multiply4/1
  Matrix Concatenate7/1 -> [row3bb]
  Constant6/1 -> Matrix Concatenate7/3
  [bb2] -> Matrix Concatenate5/3
  [bb3] -> Multiply3/1
  [bb3] -> Matrix Concatenate6/1
  [bb2] -> Multiply5/1
  Matrix Concatenate6/1 -> [row2bb]
  [row1bb] -> Matrix Concatenate8/1
  Matrix Concatenate8/1 -> [mat_xb]
  [row2bb] -> Matrix Concatenate8/2
  [row3bb] -> Matrix Concatenate8/3
  3x3 0 matrix1/1 -> Matrix Concatenate9/2
  Matrix Concatenate9/1 -> Matrix Concatenate10/2
  [mat_xb] -> Matrix Concatenate9/1
  Matrix Concatenate4/1 -> Matrix Concatenate10/1
  Matrix Concatenate10/1 -> H/1

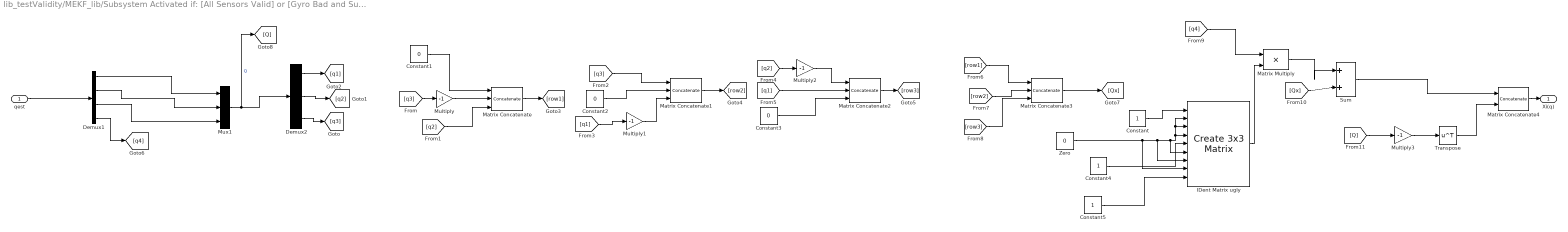
== system lib_testValidity/MEKF_lib/Subsystem Activated if: [All Sensors Valid] or [Gyro Bad and Sun//Mag sensors Valid]/Kalman Gain/Makes Xi(q) Matrix ==
  qest : Inport
  Constant : Constant
  Constant1 : Constant  Value=0
  Constant2 : Constant  Value=0
  Constant3 : Constant  Value=0
  Constant4 : Constant
  Constant5 : Constant
  Demux1 : Demux
  Demux2 : Demux  Outputs=3
  IDent Matrix ugly : sharedutil/Create 3x3 Matrix  aMode=aMode
  Matrix Concatenate : Concatenate  NumInputs=3  Mode=Multidimensional array  ConcatenateDimension=2
  Matrix Concatenate1 : Concatenate  NumInputs=3  Mode=Multidimensional array  ConcatenateDimension=2
  Matrix Concatenate2 : Concatenate  NumInputs=3  Mode=Multidimensional array  ConcatenateDimension=2
  Matrix Concatenate3 : Concatenate  NumInputs=3  Mode=Multidimensional array
  Matrix Concatenate4 : Concatenate  Mode=Multidimensional array
  Matrix Multiply : Product  Inputs=**
  Multiply{,1..3} (4 alike) : Gain  Gain=-1
  Mux1 : Mux  Inputs=3
  Sum : Sum  Inputs=|++
  Transpose : Math  Operator=transpose  SaturateOnIntegerOverflow=on
  Zero : Constant  Value=0  OutDataTypeStr=Inherit: Inherit via back propagation
  Xi(q) : Outport
  wires:
  Multiply2/1 -> Matrix Concatenate2/1
  [q1] -> Matrix Concatenate2/2
  Matrix Multiply/1 -> Sum/1
  Matrix Concatenate1/1 -> [row2]
  Constant1/1 -> Matrix Concatenate/1
  Matrix Concatenate3/1 -> [Qx]
  [q2] -> Matrix Concatenate/3
  Mux1/1 -> Demux2/1, [Q]  "Q"
  Constant2/1 -> Matrix Concatenate1/2
  Demux1/2 -> Mux1/2
  [row3] -> Matrix Concatenate3/3
  qest/1 -> Demux1/1
  Multiply3/1 -> Transpose/1
  [q4] -> Matrix Multiply/1
  [q3] -> Matrix Concatenate1/1
  Demux2/2 -> [q2]
  Sum/1 -> Matrix Concatenate4/1
  [q2] -> Multiply2/1
  Demux1/4 -> [q4]
  [row2] -> Matrix Concatenate3/2
  Demux1/1 -> Mux1/1
  Demux1/3 -> Mux1/3
  Matrix Concatenate2/1 -> [row3]
  [Qx] -> Sum/2
  Multiply/1 -> Matrix Concatenate/2
  [row1] -> Matrix Concatenate3/1
  [Q] -> Multiply3/1
  Demux2/1 -> [q1]
  Transpose/1 -> Matrix Concatenate4/2
  IDent Matrix ugly/1 -> Matrix Multiply/2
  [q3] -> Multiply/1
  Matrix Concatenate/1 -> [row1]
  Demux2/3 -> [q3]
  Constant3/1 -> Matrix Concatenate2/3
  [q1] -> Multiply1/1
  Multiply1/1 -> Matrix Concatenate1/3
  Matrix Concatenate4/1 -> Xi(q)/1
  Constant/1 -> IDent Matrix ugly/1
  Constant5/1 -> IDent Matrix ugly/9
  Constant4/1 -> IDent Matrix ugly/5
  Zero/1 -> IDent Matrix ugly/8, IDent Matrix ugly/7, IDent Matrix ugly/6, IDent Matrix ugly/4, IDent Matrix ugly/3, IDent Matrix ugly/2

== system lib_testValidity/MEKF_lib/Subsystem Activated if: [All Sensors Valid] or [Gyro Bad and Sun//Mag sensors Valid]/MEASUREMENT UPDATE TO q AND COVARIANCE2/Normalize_q ==
  note: Rearrange_Quat
  note: Rearrange_Quat_back
  Estimated Quaternion : Inport
  Demux : Demux
  Demux1 : Demux
  Mux : Mux
  Mux1 : Mux
  Quaternion Normalize : sharedutil/Quaternion Normalize  aMode=aMode
      settings: SourceProductName=Aerospace Blockset  SourceProductBaseCode=AE
  q_normalized : Outport
  wires:
  Mux1/1 -> Quaternion Normalize/1
  Demux1/4 -> Mux1/1
  Demux/4 -> Mux/3
  Demux/3 -> Mux/2
  Demux/2 -> Mux/1
  Demux1/3 -> Mux1/4
  Mux/1 -> q_normalized/1
  Demux1/1 -> Mux1/2
  Demux1/2 -> Mux1/3
  Demux/1 -> Mux/4
  Quaternion Normalize/1 -> Demux/1  "Measurement updated q estimate"
  Estimated Quaternion/1 -> Demux1/1

== system lib_testValidity/MEKF_lib/Subsystem Activated if: [All Sensors Valid] or [Gyro Bad and Sun//Mag sensors Valid]/TIME PROPAGATION of Q_EST, COVARIANCE/Psi ==
  delt : Inport
  one-half : Inport  Port=2
  om_mags : Inport  Port=3
  om_magss : Inport  Port=4
  omega_vec : Inport  Port=5
  Divide : Product  Inputs=***
  Divide1 : Product  Inputs=**/
  Sin : Trigonometry
  Psi : Outport
  wires:
  delt/1 -> Divide/1
  Divide/1 -> Sin/1  "om_mag times0.5*del_t"
  Divide1/1 -> Psi/1  "Psi"
  om_mags/1 -> Divide/3
  Sin/1 -> Divide1/1  "sin(om_mag*0.5*del_t)"
  one-half/1 -> Divide/2
  omega_vec/1 -> Divide1/2
  om_magss/1 -> Divide1/3

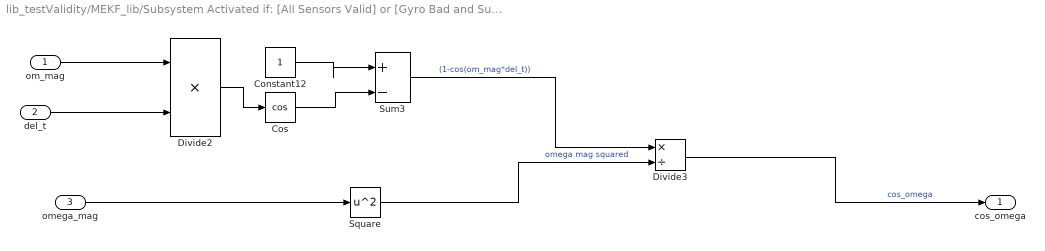
== system lib_testValidity/MEKF_lib/Subsystem Activated if: [All Sensors Valid] or [Gyro Bad and Sun//Mag sensors Valid]/TIME PROPAGATION of Q_EST, COVARIANCE/cos_omega ==
  om_mag : Inport
  del_t : Inport  Port=2
  omega_mag : Inport  Port=3
  Constant12 : Constant
  Cos : Trigonometry  Operator=cos
  Divide2 : Product  Inputs=**
  Divide3 : Product  Inputs=*/
  Square : Math  Operator=square  SaturateOnIntegerOverflow=on
  Sum3 : Sum  Inputs=|+-
  cos_omega : Outport
  wires:
  Divide2/1 -> Cos/1
  omega_mag/1 -> Square/1
  Divide3/1 -> cos_omega/1  "cos_omega"
  Constant12/1 -> Sum3/1
  Square/1 -> Divide3/2  "omega mag squared"
  om_mag/1 -> Divide2/1
  Cos/1 -> Sum3/2
  del_t/1 -> Divide2/2
  Sum3/1 -> Divide3/1  "(1-cos(om_mag*del_t))"

== system lib_testValidity/MEKF_lib/Subsystem Activated if: [Sun//Mag Sensor Invalid and Gyros are Valid] or [Gyro Invalid and Sun//Mag sensors Invalid]/TIME PROPAGATION of Q_EST, COVARIANCE/Psi ==
  In1 : Inport
  In2 : Inport  Port=2
  om_maggg : Inport  Port=3
  om_magg : Inport  Port=4
  omg_vecc : Inport  Port=5
  Divide : Product  Inputs=***
  Divide1 : Product  Inputs=**/
  Sin : Trigonometry
  Psi : Outport
  wires:
  In2/1 -> Divide/2
  Sin/1 -> Divide1/1  "sin(om_mag*0.5*del_t)"
  om_maggg/1 -> Divide/3
  Divide1/1 -> Psi/1  "Psi"
  omg_vecc/1 -> Divide1/2
  om_magg/1 -> Divide1/3
  Divide/1 -> Sin/1  "om_mag times0.5*del_t"
  In1/1 -> Divide/1

== system lib_testValidity/MEKF_lib/Subsystem Activated if: [Sun//Mag Sensor Invalid and Gyros are Valid] or [Gyro Invalid and Sun//Mag sensors Invalid]/TIME PROPAGATION of Q_EST, COVARIANCE/cos_omega ==
  In1 : Inport
  In2 : Inport  Port=2
  In3 : Inport  Port=3
  Constant12 : Constant
  Cos : Trigonometry  Operator=cos
  Divide2 : Product  Inputs=**
  Divide3 : Product  Inputs=*/
  Square : Math  Operator=square  SaturateOnIntegerOverflow=on
  Sum3 : Sum  Inputs=|+-
  cos_omega : Outport
  wires:
  Sum3/1 -> Divide3/1  "(1-cos(om_mag*del_t))"
  In2/1 -> Divide2/2
  Cos/1 -> Sum3/2
  In1/1 -> Divide2/1
  Square/1 -> Divide3/2  "omega mag squared"
  Constant12/1 -> Sum3/1
  Divide3/1 -> cos_omega/1  "cos_omega"
  In3/1 -> Square/1
  Divide2/1 -> Cos/1

== system lib_testValidity/MEKF_lib/Subsystem Activated if: [All Sensors Valid] or [Gyro Bad and Sun//Mag sensors Valid]/Kalman Gain/Create H matrix/3x3 0 matrix ==
  Create 3x3 Matrix : sharedutil/Create 3x3 Matrix  aMode=aMode
  Zero : Constant  Value=0  OutDataTypeStr=Inherit: Inherit via back propagation
  0 3x3 : Outport
  wires:
  Zero/1 -> Create 3x3 Matrix/9, Create 3x3 Matrix/8, Create 3x3 Matrix/7, Create 3x3 Matrix/6, Create 3x3 Matrix/1, Create 3x3 Matrix/5, Create 3x3 Matrix/2, Create 3x3 Matrix/3, Create 3x3 Matrix/4
  Create 3x3 Matrix/1 -> 0 3x3/1

== matlab function lib_testValidity/MEKF_lib/Subsystem Activated if: [Sun//Mag Sensor Invalid and Gyros are Valid] or [Gyro Invalid and Sun//Mag sensors Invalid]/TIME PROPAGATION of Q_EST, COVARIANCE/MATLAB Function ==
  data: omega_est input; om_mag output
function om_mag = om2_norm(omega_est)

om_mag = norm(omega_est);

== matlab function lib_testValidity/MEKF_lib/Subsystem Activated if: [Sun//Mag Sensor Invalid and Gyros are Valid] or [Gyro Invalid and Sun//Mag sensors Invalid]/TIME PROPAGATION of Q_EST, COVARIANCE/MATLAB Function10 ==
  data: del_t input; cos_omega input; om_mag input; omega_x input; State_Trans_matrix output
function State_Trans_matrix = Phi_disc(del_t,cos_omega,om_mag,omega_x)
%#codegen

State_Trans_matrix = [(eye(3)-omega_x*sin(om_mag*del_t)/om_mag + (omega_x^2)*cos_omega),omega_x*cos_omega-eye(3)*del_t-omega_x^2*(om_mag*del_t-sin(om_mag*del_t))/om_mag^3;
            zeros(3,3),eye(3)];

== matlab function lib_testValidity/MEKF_lib/Subsystem Activated if: [All Sensors Valid] or [Gyro Bad and Sun//Mag sensors Valid]/Kalman Gain/MATLAB Function2 ==
  data: R_sq input; P_sq input; H input; P_sq output; K output
function [P_sq,K] = fcnAQR(R_sq,P_sq,H)
%#codegen
[nr,mr] = size(R_sq);
[np,mp] = size(P_sq);
% A_QR = [R_sq',zeros(nr,np);(P_sq')*H', P_sq'];
A_QR = [R_sq',zeros(nr,np);(P_sq')*H', P_sq];
[TA,UA] = qr(A_QR);
        P_sq = UA(7:12,7:12)'; %Updated P_sq
        W = UA(1:6,7:12)';
%        
        sq_Bk = UA(1:6,1:6)';
K = W*inv(sq_Bk);

== matlab function lib_testValidity/MEKF_lib/Subsystem Activated if: [Sun//Mag Sensor Invalid and Gyros are Valid] or [Gyro Invalid and Sun//Mag sensors Invalid]/TIME PROPAGATION of Q_EST, COVARIANCE/MATLAB Function11 ==
  data: Phi_discrete input; P_sq output; Q_sq input; P_sq input
function P_sq  = Cqr(Phi_discrete,Q_sq,P_sq)
%#codegen

C = [P_sq'*Phi_discrete';Q_sq'];
          [Tc,Uc] = qr(C);
%           Uc = full(Uc);
          sq_P_kp1 = Uc(1:6,1:6)';
%           P = sq_P_kp1'*sq_P_kp1;
          P_sq = sq_P_kp1;

== matlab function lib_testValidity/MEKF_lib/Subsystem Activated if: [Sun//Mag Sensor Invalid and Gyros are Valid] or [Gyro Invalid and Sun//Mag sensors Invalid]/TIME PROPAGATION of Q_EST, COVARIANCE/MATLAB Function2 ==
  data: u input; om_mag output
function om_mag = norm_check1(u)
%#codegen
if u == 0
    om_mag = 10^-10;
else
    om_mag = u;
end

end

== matlab function lib_testValidity/MEKF_lib/Subsystem Activated if: [Sun//Mag Sensor Invalid and Gyros are Valid] or [Gyro Invalid and Sun//Mag sensors Invalid]/TIME PROPAGATION of Q_EST, COVARIANCE/MATLAB Function7 ==
  data: Psi input; Psi_cross output
function Psi_cross = Psi_cross_matrix(Psi)
%#codegen

Psi_cross = [0 -Psi(3) Psi(2);Psi(3) 0 -Psi(1);-Psi(2) Psi(1) 0];

== matlab function lib_testValidity/MEKF_lib/Subsystem Activated if: [Sun//Mag Sensor Invalid and Gyros are Valid] or [Gyro Invalid and Sun//Mag sensors Invalid]/TIME PROPAGATION of Q_EST, COVARIANCE/MATLAB Function8 ==
  data: Psi_x input; Psi input; om_mag input; del_t input; Omega_omega output
function Omega_omega = omega_omega_matrix(Psi_x,Psi,om_mag,del_t)
%#codegen

 Omega_omega = [(cos(0.5*om_mag*del_t)*eye(3) - Psi_x), Psi; -Psi', cos(0.5*om_mag*del_t)];

== matlab function lib_testValidity/MEKF_lib/Subsystem Activated if: [All Sensors Valid] or [Gyro Bad and Sun//Mag sensors Valid]/TIME PROPAGATION of Q_EST, COVARIANCE/MATLAB Function7 ==
  data: Psi input; Psi_cross output
function Psi_cross = Psi_cross_matrix(Psi)
%#codegen

Psi_cross = [0 -Psi(3) Psi(2);Psi(3) 0 -Psi(1);-Psi(2) Psi(1) 0];

== matlab function lib_testValidity/MEKF_lib/Subsystem Activated if: [All Sensors Valid] or [Gyro Bad and Sun//Mag sensors Valid]/TIME PROPAGATION of Q_EST, COVARIANCE/MATLAB Function8 ==
  data: Psi_x input; Psi input; om_mag input; del_t input; Omega_omega output
function Omega_omega = omega_omega_matrix(Psi_x,Psi,om_mag,del_t)
%#codegen

 Omega_omega = [(cos(0.5*om_mag*del_t)*eye(3) - Psi_x), Psi; -Psi', cos(0.5*om_mag*del_t)];

== matlab function lib_testValidity/MEKF_lib/Subsystem Activated if: [All Sensors Valid] or [Gyro Bad and Sun//Mag sensors Valid]/TIME PROPAGATION of Q_EST, COVARIANCE/MATLAB Function9 ==
  data: omega input; omega_cross_matrix output
function omega_cross_matrix = makes_omega_cross_matrix(omega)

omega_cross_matrix = [0 -omega(3) omega(2);omega(3) 0 -omega(1);-omega(2) omega(1) 0];

== matlab function lib_testValidity/MEKF_lib/Subsystem Activated if: [All Sensors Valid] or [Gyro Bad and Sun//Mag sensors Valid]/TIME PROPAGATION of Q_EST, COVARIANCE/MATLAB Function10 ==
  data: del_t input; cos_omega input; om_mag input; omega_x input; State_Trans_matrix output
function State_Trans_matrix = Phi_disc(del_t,cos_omega,om_mag,omega_x)
%#codegen

State_Trans_matrix = [(eye(3)-omega_x*sin(om_mag*del_t)/om_mag + (omega_x^2)*cos_omega),...
    omega_x*cos_omega-eye(3)*del_t-omega_x^2*(om_mag*del_t-sin(om_mag*del_t))/om_mag^3;
            zeros(3,3),eye(3)];

== matlab function lib_testValidity/MEKF_lib/Subsystem Activated if: [All Sensors Valid] or [Gyro Bad and Sun//Mag sensors Valid]/TIME PROPAGATION of Q_EST, COVARIANCE/MATLAB Function11 ==
  data: Phi_discrete input; P_sq output; Q_sq input; P_sq input
function P_sq  = Cqr(Phi_discrete,Q_sq,P_sq)
%#codegen

C = [P_sq'*Phi_discrete';Q_sq'];
          [Tc,Uc] = qr(C);
%           Uc = full(Uc);
          sq_P_kp1 = Uc(1:6,1:6)';
%           P = sq_P_kp1'*sq_P_kp1;
          P_sq = sq_P_kp1;

== matlab function lib_testValidity/MEKF_lib/Subsystem Activated if: [Sun//Mag Sensor Invalid and Gyros are Valid] or [Gyro Invalid and Sun//Mag sensors Invalid]/TIME PROPAGATION of Q_EST, COVARIANCE/MATLAB Function9 ==
  data: omega input; omega_cross_matrix output
function omega_cross_matrix = makes_omega_cross_matrix(omega)

omega_cross_matrix = [0 -omega(3) omega(2);omega(3) 0 -omega(1);-omega(2) omega(1) 0];

== matlab function lib_testValidity/MEKF_lib/Subsystem Activated if: [All Sensors Valid] or [Gyro Bad and Sun//Mag sensors Valid]/MEASUREMENT UPDATE TO q AND COVARIANCE2/MATLAB Function ==
  data: qe input; qe_n output
function qe_n = fcn(qe)
%#codegen

qe_n = 1/(norm(qe))*qe;

== matlab function lib_testValidity/MEKF_lib/Subsystem Activated if: [All Sensors Valid] or [Gyro Bad and Sun//Mag sensors Valid]/TIME PROPAGATION of Q_EST, COVARIANCE/MATLAB Function ==
  data: omega_est input; om_mag output
function om_mag = om2_norm(omega_est)

om_mag = norm(omega_est);

== matlab function lib_testValidity/MEKF_lib/Subsystem Activated if: [All Sensors Valid] or [Gyro Bad and Sun//Mag sensors Valid]/Kalman Gain/MATLAB Function ==
  data: rb_hat input; H output size=[6,6]; bhat input
function H  = fcn(rb_hat,bhat)
%#codegen

            mat_x = [0 -rb_hat(3) rb_hat(2);rb_hat(3) 0 -rb_hat(1);-rb_hat(2) rb_hat(1) 0]; %cross product matrix of q
            mat_x1 = [0 -bhat(3) bhat(2);bhat(3) 0 -bhat(1);-bhat(2) bhat(1) 0];
        
%%%%% Calcualte Kalman Gain
        H = [mat_x, zeros(3,3);mat_x1,zeros(3,3)]; %sensitivity matrix'

== matlab function lib_testValidity/MEKF_lib/Subsystem Activated if: [All Sensors Valid] or [Gyro Bad and Sun//Mag sensors Valid]/TIME PROPAGATION of Q_EST, COVARIANCE/MATLAB Function2 ==
  data: u input; om_mag output
function om_mag = norm_check1(u)
%#codegen
if u == 0
    om_mag = 10^-10;
else
    om_mag = u;
end
end

== matlab function lib_testValidity/MEKF_lib/Subsystem Activated if: [All Sensors Valid] or [Gyro Bad and Sun//Mag sensors Valid]/Kalman Gain/MATLAB Function1 ==
  data: qe input; Xi_q output
function Xi_q = fcn(qe)
%#codegen

Q = [qe(1:3,1)];
            Qx = [0 -qe(3) qe(2);qe(3) 0 -qe(1);-qe(2) qe(1) 0]; %cross product matrix of q
                Xi_q = [qe(4)*eye(3)+Qx;-Q'];
